simulink model "simulation_projet"  (R2019a)
settings: Solver=VariableStepAuto  StartTime=0.0  StopTime=Tsim  RelTol=1e-3
values from neighbouring files (symbols this model uses):
  F1 = 85005.9    [Simulation_projet.m]
  F2 = 90000    [Simulation_projet.m]
  F3 = 94986.8    [Simulation_projet.m]
  F4 = 100000    [Simulation_projet.m]
  F5 = 115015.9    [Simulation_projet.m]
  F6 = 120000    [Simulation_projet.m]
  Te = 1/Fe    (= 3.125e-06)    [Simulation_projet.m]    (also in script_matlab.m = 0.03125)
settings Model: Creator=dechambe  LastModifiedBy=dechambe

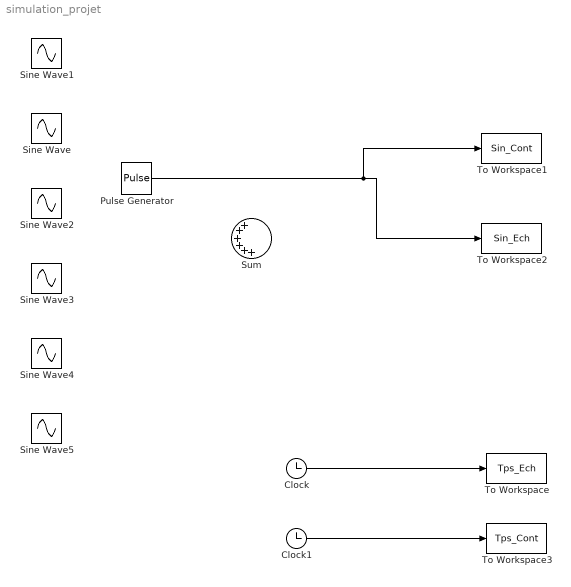
== system simulation_projet ==
  Clock : Clock
  Clock1 : Clock
  Pulse Generator : DiscretePulseGenerator  PulseType=Time based  Period=1/85000  PulseWidth=50
  Sine Wave : Sin  Frequency=F2*2*pi()  SampleTime=0
  Sine Wave1 : Sin  Frequency=F1*2*pi()  SampleTime=0
  Sine Wave2 : Sin  Frequency=F3*2*pi()  SampleTime=0
  Sine Wave3 : Sin  Frequency=F4*2*pi()  SampleTime=0
  Sine Wave4 : Sin  Frequency=F5*2*pi()  SampleTime=0
  Sine Wave5 : Sin  Frequency=F6*2*pi()  SampleTime=0
  Sum : Sum  Inputs=|++++++
  To Workspace : ToWorkspace  VariableName=Tps_Ech  SampleTime=Te
      settings: Save2DSignal=2-D array (concatenate along first dimension)
  To Workspace1 : ToWorkspace  VariableName=Sin_Cont  SampleTime=Te/100
      settings: Save2DSignal=2-D array (concatenate along first dimension)
  To Workspace2 : ToWorkspace  VariableName=Sin_Ech  SampleTime=Te
      settings: Save2DSignal=2-D array (concatenate along first dimension)
  To Workspace3 : ToWorkspace  VariableName=Tps_Cont  SampleTime=Te/100
      settings: Save2DSignal=2-D array (concatenate along first dimension)
  wires:
  Clock1/1 -> To Workspace3/1
  Clock/1 -> To Workspace/1
  Pulse Generator/1 -> To Workspace1/1, To Workspace2/1
